simulink model "Kettle_System2_1"  (R2017b)
settings: Solver=VariableStepAuto  StartTime=0.0  StopTime=1000  FixedStep=1  MaxStep=1  RelTol=1e-3
libraries: simulink_extras x1
settings Model: DataTypeOverride=Double  MinMaxOverflowLogging=ForceOff  Creator=georgimarkov & jonhall  LastModifiedBy=georgimarkov

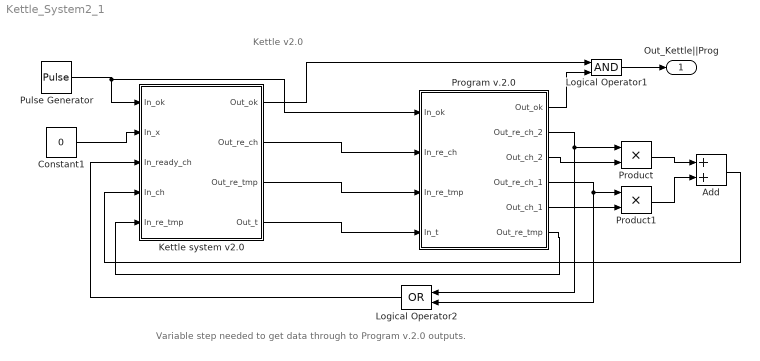
== system Kettle_System2_1 ==
  note: Variable step needed to get data through to Program v.2.0 outputs.
  note: Kettle v2.0
  Add : Sum
  Constant1 : Constant  Value=0
  Kettle system v2.0 : Subsystem
  Logical Operator1 : Logic  AllPortsSameDT=off  OutDataTypeStr=boolean
  Logical Operator2 : Logic  Operator=OR  AllPortsSameDT=off  OutDataTypeStr=boolean
  Product : Product
  Product1 : Product
  Program v.2.0 : Subsystem
  Pulse Generator : DiscretePulseGenerator  Period=200  PhaseDelay=10
  Out_Kettle||Prog : Outport
  wires:
  Program v.2.0/1(Out_ok) -> Logical Operator1/2
  Kettle system v2.0/1(Out_ok) -> Logical Operator1/1
  Logical Operator1/1 -> Out_Kettle||Prog/1
  Constant1/1 -> Kettle system v2.0/2(In_x)
  Kettle system v2.0/2(Out_re_ch) -> Program v.2.0/2(In_re_ch)
  Kettle system v2.0/3(Out_re_tmp) -> Program v.2.0/3(In_re_tmp)
  Program v.2.0/2(Out_re_ch_2) -> Logical Operator2/1, Product/1
  Program v.2.0/3(Out_ch_2) -> Product/2
  Program v.2.0/4(Out_re_ch_1) -> Logical Operator2/2, Product1/1
  Program v.2.0/5(Out_ch_1) -> Product1/2
  Product/1 -> Add/1
  Product1/1 -> Add/2
  Add/1 -> Kettle system v2.0/4(In_ch)
  Program v.2.0/6(Out_re_tmp) -> Kettle system v2.0/5(In_re_tmp)
  Logical Operator2/1 -> Kettle system v2.0/3(In_ready_ch)
  Kettle system v2.0/4(Out_t) -> Program v.2.0/4(In_t)
  Pulse Generator/1 -> Program v.2.0/1(In_ok), Kettle system v2.0/1(In_ok)

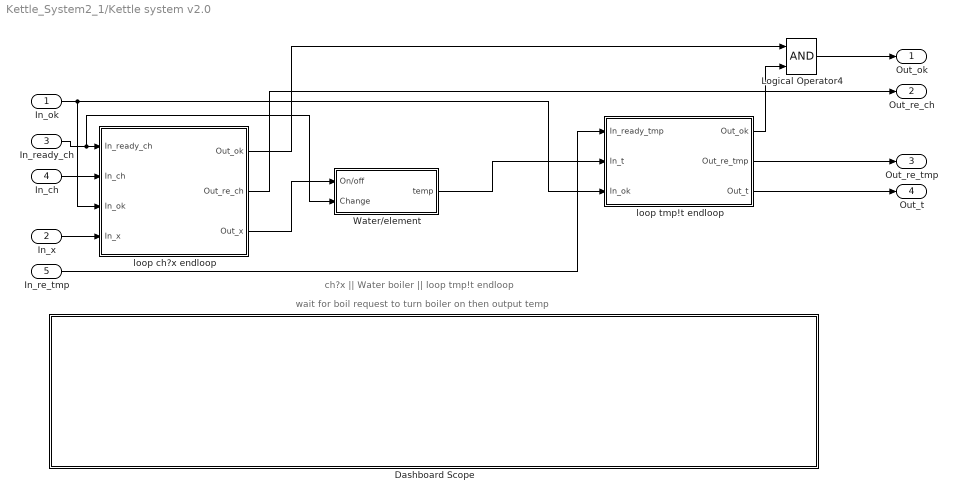
== system Kettle_System2_1/Kettle system v2.0 ==
  note: ch?x || Water boiler || loop tmp!t endloop
  note: wait for boil request to turn boiler on then output temp
  In_ok : Inport
  In_x : Inport  Port=2
  In_ready_ch : Inport  Port=3
  In_ch : Inport  Port=4
  In_re_tmp : Inport  Port=5
  Dashboard Scope : Subsystem  DialogController=hmiCreateDDGDialog  IsWebBlock=on  mask(MWDashboardBlock){webBlockId=0c6ab515-e131-4fbc-9890-d7af2ac4fa79, webBlockType=sdiscope, ShowInitialText=on, HMISrcModelName=Kettle_System2_1}
      mask prompts: webBlockId "WebBlock Id"; webBlockType "WebBlock Type"; HMISrcModelName "Source Model"
      mask help: SimulinkHMI:dialogs:HMIScopeDialogDesc
      mask Help: helpview([docroot '/mapfiles/simulink.map'], 'hmi_scope')
      mask Display:
      | if strcmp(get_param(bdroot(gcb),'BlockDiagramType'), 'library')
      |     image([(matlabroot) '/toolbox/simulink/hmi/icons/DashboardScope.png']);
      | end
  Logical Operator4 : Logic  AllPortsSameDT=off  OutDataTypeStr=fixdt(1,16)
  Water/element : Subsystem  TreatAsAtomicUnit=on  SystemSampleTime=0
  loop ch?x endloop : Subsystem
  loop tmp!t endloop : Subsystem
  Out_ok : Outport
  Out_re_ch : Outport  Port=2
  Out_re_tmp : Outport  Port=3
  Out_t : Outport  Port=4
  wires:
  Water/element/1(temp) -> loop tmp!t endloop/2(In_t)
  In_ok/1 -> loop tmp!t endloop/3(In_ok), loop ch?x endloop/3(In_ok)
  In_x/1 -> loop ch?x endloop/4(In_x)
  In_ready_ch/1 -> Water/element/2(Change), loop ch?x endloop/1(In_ready_ch)
  In_ch/1 -> loop ch?x endloop/2(In_ch)
  loop tmp!t endloop/1(Out_ok) -> Logical Operator4/2
  Logical Operator4/1 -> Out_ok/1
  In_re_tmp/1 -> loop tmp!t endloop/1(In_ready_tmp)
  loop tmp!t endloop/2(Out_re_tmp) -> Out_re_tmp/1
  loop tmp!t endloop/3(Out_t) -> Out_t/1
  loop ch?x endloop/1(Out_ok) -> Logical Operator4/1
  loop ch?x endloop/2(Out_re_ch) -> Out_re_ch/1
  loop ch?x endloop/3(Out_x) -> Water/element/1(On/off)

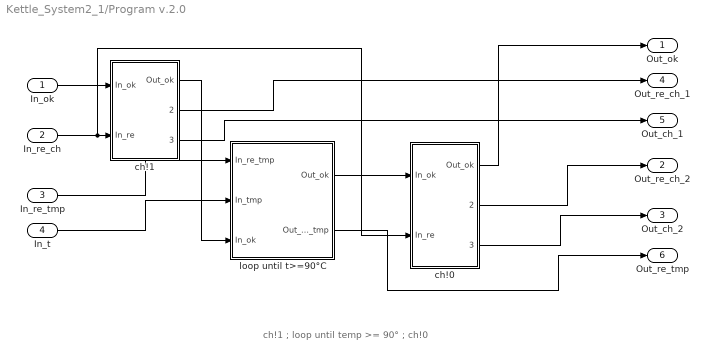
== system Kettle_System2_1/Program v.2.0 ==
  note: ch!1 ; loop until temp >= 90° ; ch!0
  In_ok : Inport
  In_re_ch : Inport  Port=2
  In_re_tmp : Inport  Port=3
  In_t : Inport  Port=4
  ch!0 : Subsystem
  "ch!1 " : Subsystem
  loop until t>=90°C : Subsystem
  Out_ok : Outport
  Out_re_ch_2 : Outport  Port=2
  Out_ch_2 : Outport  Port=3
  Out_re_ch_1 : Outport  Port=4
  Out_ch_1 : Outport  Port=5
  Out_re_tmp : Outport  Port=6
  wires:
  ch!0/2(Out_re_ch_2) -> Out_re_ch_2/1
  loop until t>=90°C/1(Out_ok) -> ch!0/1(In_ok)
  "ch!1 "/2(Out_re_ch_1) -> Out_re_ch_1/1
  "ch!1 "/1(Out_ok) -> loop until t>=90°C/3(In_ok)
  ch!0/1(Out_ok) -> Out_ok/1
  In_ok/1 -> "ch!1 "/1(In_ok)
  In_re_ch/1 -> ch!0/2(In_re), "ch!1 "/2(In_re)
  In_re_tmp/1 -> loop until t>=90°C/1(In_re_tmp)
  ch!0/3(Out_ch_2) -> Out_ch_2/1
  "ch!1 "/3("Out_ch_1 ") -> Out_ch_1/1
  loop until t>=90°C/2(Out_re_tmp) -> Out_re_tmp/1
  In_t/1 -> loop until t>=90°C/2(In_tmp)

== system Kettle_System2_1/Kettle system v2.0/Dashboard Scope ==

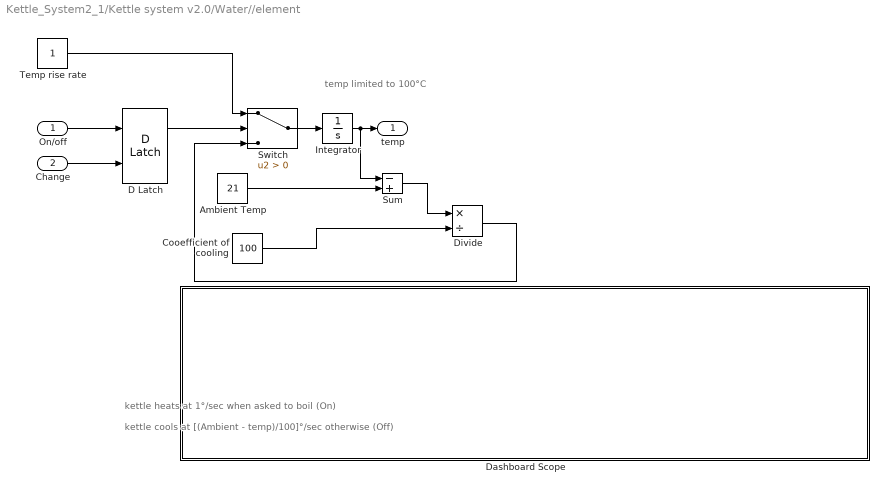
== system Kettle_System2_1/Kettle system v2.0/Water//element ==
  note: temp limited to 100°C
  note: kettle heats at 1°/sec when asked to boil (On)
  note: kettle cools at [(Ambient - temp)/100]°/sec otherwise (Off)
  On/off : Inport
  Change : Inport  Port=2
  "Ambient Temp " : Constant  Value=21
  Cooefficient of cooling : Constant  Value=100
  D Latch : simulink_extras/Flip Flops/D Latch
      settings: SourceProductName=Simulink  SourceProductBaseCode=SL
  Dashboard Scope : Subsystem  DialogController=hmiCreateDDGDialog  IsWebBlock=on  mask(MWDashboardBlock){webBlockId=a0783e22-3817-44e7-9254-d29470bf7746, webBlockType=sdiscope, ShowInitialText=on, HMISrcModelName=Kettle_System2_1}
      mask prompts: webBlockId "WebBlock Id"; webBlockType "WebBlock Type"; HMISrcModelName "Source Model"
      mask help: SimulinkHMI:dialogs:HMIScopeDialogDesc
      mask Help: helpview([docroot '/mapfiles/simulink.map'], 'hmi_scope')
      mask Display:
      | if strcmp(get_param(bdroot(gcb),'BlockDiagramType'), 'library')
      |     image([(matlabroot) '/toolbox/simulink/hmi/icons/DashboardScope.png']);
      | end
  Divide : Product  Inputs=*/
  Integrator : Integrator  InitialCondition=21  LimitOutput=on  UpperSaturationLimit=100  LowerSaturationLimit=-273.15
  Sum : Sum  Inputs=-+
  Switch : Switch  Criteria=u2 > Threshold
  Temp rise rate : Constant
  temp : Outport
  wires:
  Switch/1 -> Integrator/1
  Temp rise rate/1 -> Switch/1
  Divide/1 -> Switch/3
  D Latch/1 -> Switch/2
  Change/1 -> D Latch/2
  On/off/1 -> D Latch/1
  Integrator/1 -> Sum/1, temp/1
  Sum/1 -> Divide/1
  "Ambient Temp "/1 -> Sum/2
  Cooefficient of cooling/1 -> Divide/2

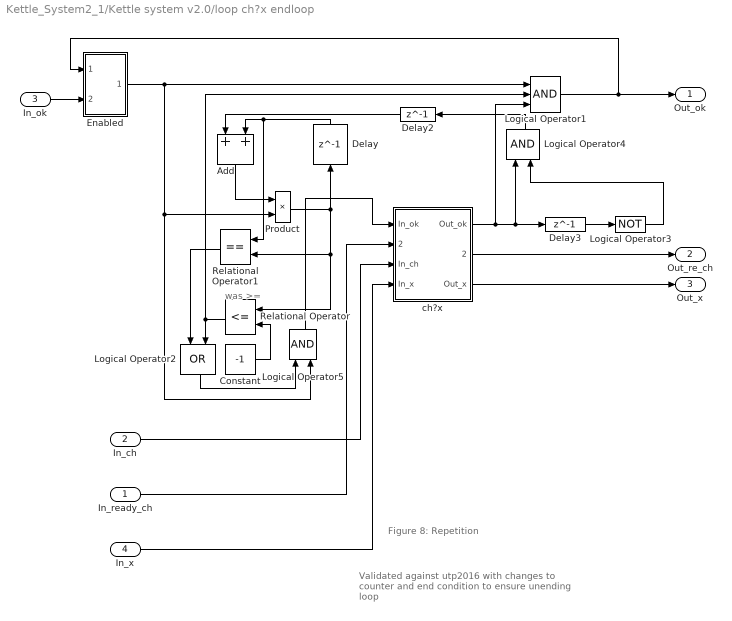
== system Kettle_System2_1/Kettle system v2.0/loop ch?x endloop ==
  note: was >=
  note: Figure 8: Repetition
  note: Validated against utp2016
      | with changes to counter and end condition to
      | ensure unending loop
  In_ready_ch : Inport
  In_ch : Inport  Port=2
  In_ok : Inport  Port=3
  In_x : Inport  Port=4
  Add : Sum
  Constant : Constant  Value=-1
  Delay : Delay  DelayLength=1  InitialCondition=0
  Delay2 : Delay  DelayLength=1  InitialCondition=0
  Delay3 : Delay  DelayLength=1  InitialCondition=0
  Enabled : Subsystem
  Logical Operator1 : Logic  Inputs=3  AllPortsSameDT=off  OutDataTypeStr=fixdt(1,16)
  Logical Operator2 : Logic  Operator=OR  AllPortsSameDT=off  OutDataTypeStr=fixdt(1,16)
  Logical Operator3 : Logic  Operator=NOT  AllPortsSameDT=off  OutDataTypeStr=fixdt(1,16)
  Logical Operator4 : Logic  AllPortsSameDT=off  OutDataTypeStr=fixdt(1,16)
  Logical Operator5 : Logic  AllPortsSameDT=off  OutDataTypeStr=fixdt(1,16)
  Product : Product
  Relational Operator : RelationalOperator  Operator=<=  OutDataTypeStr=boolean  RndMeth=Simplest
  Relational Operator1 : RelationalOperator  Operator===  OutDataTypeStr=boolean  RndMeth=Simplest
  ch?x : Subsystem
  Out_ok : Outport
  Out_re_ch : Outport  Port=2
  Out_x : Outport  Port=3
  wires:
  Enabled/1(Enabled) -> Logical Operator1/1, Product/2, Logical Operator5/2
  Logical Operator1/1 -> Enabled/1(Out_ok), Out_ok/1
  In_ch/1 -> ch?x/3(In_ch)
  Logical Operator4/1 -> Delay2/1
  Logical Operator2/1 -> Logical Operator5/1
  Delay3/1 -> Logical Operator3/1
  Constant/1 -> Relational Operator/2
  Delay2/1 -> Add/1
  Logical Operator3/1 -> Logical Operator4/2
  Delay/1 -> Add/2, Relational Operator1/1
  In_ready_ch/1 -> ch?x/2(In_re_ch)
  Add/1 -> Product/1
  Product/1 -> Relational Operator/1, Relational Operator1/2, Delay/1
  Logical Operator5/1 -> ch?x/1(In_ok)
  Relational Operator1/1 -> Logical Operator2/1
  Relational Operator/1 -> Logical Operator1/2, Logical Operator2/2
  In_ok/1 -> Enabled/2(In_ok)
  ch?x/1(Out_ok) -> Logical Operator4/1, Delay3/1, Logical Operator1/3
  ch?x/2(Out_re_ch) -> Out_re_ch/1
  ch?x/3("Out_x ") -> Out_x/1
  In_x/1 -> ch?x/4(In_x)

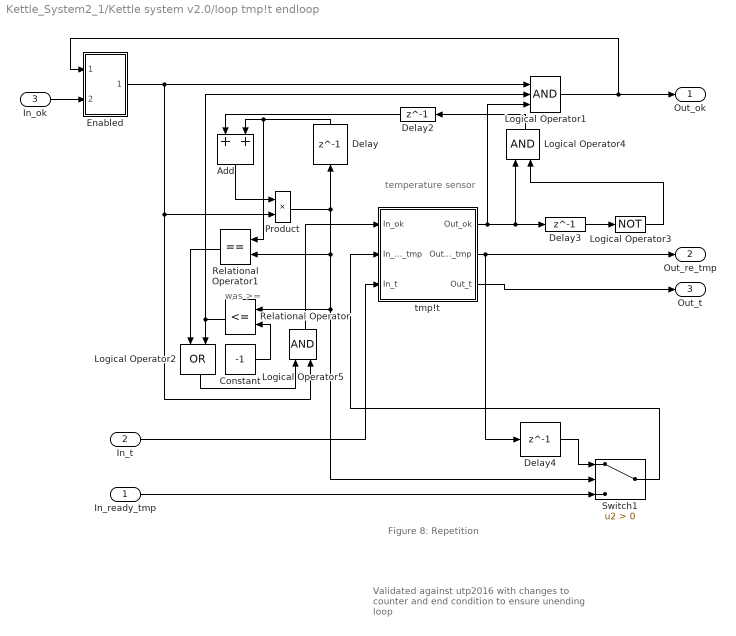
== system Kettle_System2_1/Kettle system v2.0/loop tmp!t endloop ==
  note: was >=
  note: Figure 8: Repetition
  note: temperature sensor
  note: Validated against utp2016
      | with changes to counter and end condition to
      | ensure unending loop
  In_ready_tmp : Inport
  In_t : Inport  Port=2
  In_ok : Inport  Port=3
  Add : Sum
  Constant : Constant  Value=-1
  Delay{,2..4} (4 alike) : Delay  DelayLength=1  InitialCondition=0
  Enabled : Subsystem
  Logical Operator1 : Logic  Inputs=3  AllPortsSameDT=off  OutDataTypeStr=fixdt(1,16)
  Logical Operator2 : Logic  Operator=OR  AllPortsSameDT=off  OutDataTypeStr=fixdt(1,16)
  Logical Operator3 : Logic  Operator=NOT  AllPortsSameDT=off  OutDataTypeStr=fixdt(1,16)
  Logical Operator4 : Logic  AllPortsSameDT=off  OutDataTypeStr=fixdt(1,16)
  Logical Operator5 : Logic  AllPortsSameDT=off  OutDataTypeStr=fixdt(1,16)
  Product : Product
  Relational Operator : RelationalOperator  Operator=<=  OutDataTypeStr=boolean  RndMeth=Simplest
  Relational Operator1 : RelationalOperator  Operator===  OutDataTypeStr=boolean  RndMeth=Simplest
  Switch1 : Switch  Criteria=u2 > Threshold  OutDataTypeStr=double
  tmp!t : Subsystem
  Out_ok : Outport
  Out_re_tmp : Outport  Port=2
  Out_t : Outport  Port=3
  wires:
  Enabled/1(Enabled) -> Logical Operator1/1, Product/2, Logical Operator5/2
  Logical Operator1/1 -> Enabled/1(Out_ok), Out_ok/1
  In_t/1 -> tmp!t/3(In_t)
  Logical Operator4/1 -> Delay2/1
  tmp!t/1(Out_ok) -> Delay3/1, Logical Operator4/1, Logical Operator1/3
  Logical Operator2/1 -> Logical Operator5/1
  Delay3/1 -> Logical Operator3/1
  Constant/1 -> Relational Operator/2
  tmp!t/2(Out_re_tmp) -> Out_re_tmp/1, Delay4/1
  Delay2/1 -> Add/1
  Logical Operator3/1 -> Logical Operator4/2
  Delay/1 -> Add/2, Relational Operator1/1
  In_ready_tmp/1 -> Switch1/3
  Delay4/1 -> Switch1/1
  Switch1/1 -> tmp!t/2(In_re_tmp)
  tmp!t/3("Out_t ") -> Out_t/1
  Add/1 -> Product/1
  Product/1 -> Relational Operator/1, Switch1/2, Relational Operator1/2, Delay/1
  Logical Operator5/1 -> tmp!t/1(In_ok)
  Relational Operator1/1 -> Logical Operator2/1
  Relational Operator/1 -> Logical Operator1/2, Logical Operator2/2
  In_ok/1 -> Enabled/2(In_ok)

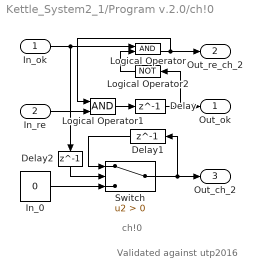
== system Kettle_System2_1/Program v.2.0/ch!0 ==
  note: Validated against utp2016
  note: ch!0
  In_ok : Inport
  In_re : Inport  Port=2
  Delay : Delay  DelayLength=1  InitialCondition=0
  Delay1 : Delay  DelayLength=1  InitialCondition=0
  Delay2 : Delay  DelayLength=1  InitialCondition=0
  "In_0 " : Constant  Value=0
  Logical Operator : Logic  AllPortsSameDT=off  OutDataTypeStr=fixdt(1,16)
  Logical Operator1 : Logic  AllPortsSameDT=off  OutDataTypeStr=fixdt(1,16)
  Logical Operator2 : Logic  Operator=NOT  AllPortsSameDT=off  OutDataTypeStr=fixdt(1,16)
  Switch : Switch  Criteria=u2 > Threshold
  Out_ok : Outport
  Out_re_ch_2 : Outport  Port=2
  Out_ch_2 : Outport  Port=3
  wires:
  In_re/1 -> Logical Operator1/2
  Logical Operator2/1 -> Logical Operator/2
  Logical Operator1/1 -> Delay/1
  In_ok/1 -> Logical Operator/1, Delay2/1
  Delay2/1 -> Switch/2
  Logical Operator/1 -> Out_re_ch_2/1, Logical Operator1/1
  Switch/1 -> Delay1/1, Out_ch_2/1
  Delay1/1 -> Switch/1
  "In_0 "/1 -> Switch/3
  Delay/1 -> Out_ok/1, Logical Operator2/1

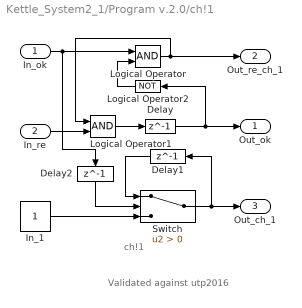
== system Kettle_System2_1/Program v.2.0/ch!1  ==
  note: Validated against utp2016
  note: ch!1
  In_ok : Inport
  In_re : Inport  Port=2
  Delay : Delay  DelayLength=1  InitialCondition=0
  Delay1 : Delay  DelayLength=1  InitialCondition=0
  Delay2 : Delay  DelayLength=1  InitialCondition=0
  In_1 : Constant
  Logical Operator : Logic  AllPortsSameDT=off  OutDataTypeStr=fixdt(1,16)
  Logical Operator1 : Logic  AllPortsSameDT=off  OutDataTypeStr=fixdt(1,16)
  Logical Operator2 : Logic  Operator=NOT  AllPortsSameDT=off  OutDataTypeStr=boolean
  Switch : Switch  Criteria=u2 > Threshold
  Out_ok : Outport
  Out_re_ch_1 : Outport  Port=2
  "Out_ch_1 " : Outport  Port=3
  wires:
  In_re/1 -> Logical Operator1/2
  Logical Operator2/1 -> Logical Operator/2
  In_ok/1 -> Delay2/1, Logical Operator/1
  Delay2/1 -> Switch/2
  Switch/1 -> Delay1/1, "Out_ch_1 "/1
  Delay1/1 -> Switch/1
  In_1/1 -> Switch/3
  Logical Operator/1 -> Out_re_ch_1/1, Logical Operator1/1
  Logical Operator1/1 -> Delay/1
  Delay/1 -> Logical Operator2/1, Out_ok/1

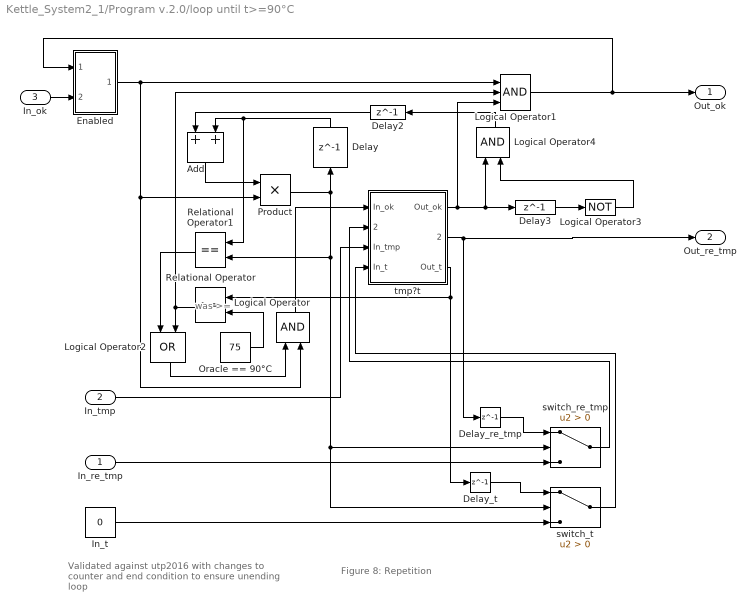
== system Kettle_System2_1/Program v.2.0/loop until t>=90°C ==
  note: Figure 8: Repetition
  note: was >=
  note: Validated against utp2016
      | with changes to counter and end condition to
      | ensure unending loop
  In_re_tmp : Inport
  In_tmp : Inport  Port=2
  In_ok : Inport  Port=3
  Add : Sum
  Delay : Delay  DelayLength=1  InitialCondition=0
  Delay2 : Delay  DelayLength=1  InitialCondition=0
  Delay3 : Delay  DelayLength=1  InitialCondition=0
  Delay_re_tmp : Delay  DelayLength=1  InitialCondition=0
  Delay_t : Delay  DelayLength=1  InitialCondition=0
  Enabled : Subsystem
  In_t : Constant  Value=0
  Logical Operator : Logic  AllPortsSameDT=off  OutDataTypeStr=boolean
  Logical Operator1 : Logic  Inputs=3  AllPortsSameDT=off  OutDataTypeStr=fixdt(1,16)
  Logical Operator2 : Logic  Operator=OR  AllPortsSameDT=off  OutDataTypeStr=fixdt(1,16)
  Logical Operator3 : Logic  Operator=NOT  AllPortsSameDT=off  OutDataTypeStr=fixdt(1,16)
  Logical Operator4 : Logic  AllPortsSameDT=off  OutDataTypeStr=fixdt(1,16)
  Oracle == 90°C : Constant  Value=75
  Product : Product
  Relational Operator : RelationalOperator  OutDataTypeStr=boolean  RndMeth=Simplest
  Relational Operator1 : RelationalOperator  Operator===  OutDataTypeStr=boolean  RndMeth=Simplest
  switch_re_tmp : Switch  Criteria=u2 > Threshold  OutDataTypeStr=double
  switch_t : Switch  Criteria=u2 > Threshold  OutDataTypeStr=double
  tmp?t : Subsystem
  Out_ok : Outport
  Out_re_tmp : Outport  Port=2
  wires:
  Enabled/1(Enabled) -> Logical Operator/2, Product/2, Logical Operator1/1
  In_tmp/1 -> tmp?t/3(In_tmp)
  Oracle == 90°C/1 -> Relational Operator/2
  Delay_t/1 -> switch_t/1
  Logical Operator3/1 -> Logical Operator4/2
  Logical Operator1/1 -> Enabled/1(Out_ok), Out_ok/1
  Relational Operator/1 -> Logical Operator2/2, Logical Operator1/2
  Delay/1 -> Add/2, Relational Operator1/1
  In_re_tmp/1 -> switch_re_tmp/3
  Logical Operator4/1 -> Delay2/1
  Delay2/1 -> Add/1
  tmp?t/3("Out_t ") -> Delay_t/1, Relational Operator/1
  tmp?t/1(Out_ok) -> Delay3/1, Logical Operator4/1, Logical Operator1/3
  Delay3/1 -> Logical Operator3/1
  tmp?t/2(Out_re_tmp) -> Out_re_tmp/1, Delay_re_tmp/1
  In_t/1 -> switch_t/3
  switch_re_tmp/1 -> tmp?t/2(In_re_tmp)
  switch_t/1 -> tmp?t/4(In_t)
  Delay_re_tmp/1 -> switch_re_tmp/1
  Relational Operator1/1 -> Logical Operator2/1
  Logical Operator2/1 -> Logical Operator/1
  Logical Operator/1 -> tmp?t/1(In_ok)
  Add/1 -> Product/1
  Product/1 -> switch_t/2, switch_re_tmp/2, Relational Operator1/2, Delay/1
  In_ok/1 -> Enabled/2(In_ok)

== system Kettle_System2_1/Kettle system v2.0/Water//element/Dashboard Scope ==

== system Kettle_System2_1/Kettle system v2.0/loop ch?x endloop/Enabled ==
  Out_ok : Inport
  In_ok : Inport  Port=2
  Delay : Delay  DelayLength=1  InitialCondition=0
  Delay1 : Delay  DelayLength=1  InitialCondition=0
  Logical Operator : Logic  Operator=OR  AllPortsSameDT=off  OutDataTypeStr=boolean
  Logical Operator1 : Logic  Operator=NOT  AllPortsSameDT=off  OutDataTypeStr=boolean
  Logical Operator2 : Logic  AllPortsSameDT=off  OutDataTypeStr=boolean
  Logical Operator3 : Logic  AllPortsSameDT=off  OutDataTypeStr=boolean
  Logical Operator4 : Logic  Operator=NOT  AllPortsSameDT=off  OutDataTypeStr=boolean
  Enabled : Outport
  wires:
  Logical Operator/1 -> Delay/1, Enabled/1
  Delay/1 -> Logical Operator3/2, Logical Operator1/1
  In_ok/1 -> Logical Operator2/1
  Logical Operator1/1 -> Logical Operator2/2
  Logical Operator2/1 -> Logical Operator/2
  Out_ok/1 -> Delay1/1
  Logical Operator3/1 -> Logical Operator/1
  Delay1/1 -> Logical Operator4/1
  Logical Operator4/1 -> Logical Operator3/1

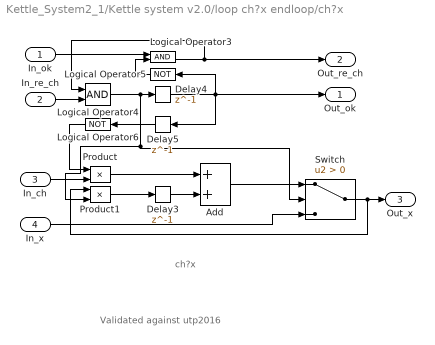
== system Kettle_System2_1/Kettle system v2.0/loop ch?x endloop/ch?x ==
  note: Validated against utp2016
  note: ch?x
  In_ok : Inport
  In_re_ch : Inport  Port=2
  In_ch : Inport  Port=3
  In_x : Inport  Port=4
  Add : Sum
  Delay3 : Delay  DelayLength=1  InitialCondition=0
  Delay4 : Delay  DelayLength=1  InitialCondition=0
  Delay5 : Delay  DelayLength=1  InitialCondition=0
  Logical Operator3 : Logic  AllPortsSameDT=off  OutDataTypeStr=fixdt(1,16)
  Logical Operator4 : Logic  AllPortsSameDT=off  OutDataTypeStr=fixdt(1,16)
  Logical Operator5 : Logic  Operator=NOT  AllPortsSameDT=off  OutDataTypeStr=fixdt(1,16)
  Logical Operator6 : Logic  Operator=NOT  AllPortsSameDT=off  OutDataTypeStr=fixdt(1,16)
  Product : Product
  Product1 : Product
  Switch : Switch  Criteria=u2 > Threshold
  Out_ok : Outport
  Out_re_ch : Outport  Port=2
  "Out_x " : Outport  Port=3
  wires:
  In_ch/1 -> Product/2
  In_ok/1 -> Logical Operator3/1
  Delay4/1 -> Out_ok/1, Delay5/1, Logical Operator5/1
  Product1/1 -> Delay3/1
  In_re_ch/1 -> Logical Operator4/2
  Logical Operator5/1 -> Logical Operator3/2
  Product/1 -> Add/1
  Delay3/1 -> Add/2
  Logical Operator6/1 -> Product/1
  Add/1 -> Switch/1
  Delay5/1 -> Logical Operator6/1
  Logical Operator3/1 -> Out_re_ch/1, Logical Operator4/1
  In_x/1 -> Switch/3
  Switch/1 -> "Out_x "/1, Product1/1
  Logical Operator4/1 -> Product1/2, Switch/2, Delay4/1

== system Kettle_System2_1/Kettle system v2.0/loop tmp!t endloop/Enabled ==
  Out_ok : Inport
  In_ok : Inport  Port=2
  Delay : Delay  DelayLength=1  InitialCondition=0
  Delay1 : Delay  DelayLength=1  InitialCondition=0
  Logical Operator : Logic  Operator=OR  AllPortsSameDT=off  OutDataTypeStr=boolean
  Logical Operator1 : Logic  Operator=NOT  AllPortsSameDT=off  OutDataTypeStr=boolean
  Logical Operator2 : Logic  AllPortsSameDT=off  OutDataTypeStr=boolean
  Logical Operator3 : Logic  AllPortsSameDT=off  OutDataTypeStr=boolean
  Logical Operator4 : Logic  Operator=NOT  AllPortsSameDT=off  OutDataTypeStr=boolean
  Enabled : Outport
  wires:
  Logical Operator/1 -> Delay/1, Enabled/1
  Delay/1 -> Logical Operator3/2, Logical Operator1/1
  In_ok/1 -> Logical Operator2/1
  Logical Operator1/1 -> Logical Operator2/2
  Logical Operator2/1 -> Logical Operator/2
  Out_ok/1 -> Delay1/1
  Logical Operator3/1 -> Logical Operator/1
  Delay1/1 -> Logical Operator4/1
  Logical Operator4/1 -> Logical Operator3/1

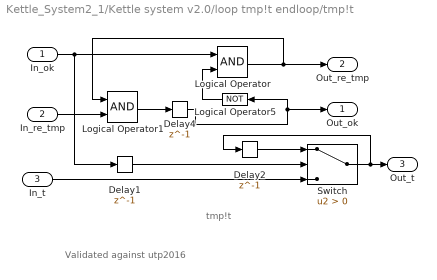
== system Kettle_System2_1/Kettle system v2.0/loop tmp!t endloop/tmp!t ==
  note: Validated against utp2016
  note: tmp!t
  In_ok : Inport
  In_re_tmp : Inport  Port=2
  In_t : Inport  Port=3
  Delay1 : Delay  DelayLength=1  InitialCondition=0
  Delay2 : Delay  DelayLength=1  InitialCondition=0
  Delay4 : Delay  DelayLength=1  InitialCondition=0
  Logical Operator : Logic  AllPortsSameDT=off  OutDataTypeStr=boolean
  Logical Operator1 : Logic  AllPortsSameDT=off  OutDataTypeStr=boolean
  Logical Operator5 : Logic  Operator=NOT  AllPortsSameDT=off  OutDataTypeStr=fixdt(1,16)
  Switch : Switch  Criteria=u2 > Threshold
  Out_ok : Outport
  Out_re_tmp : Outport  Port=2
  "Out_t " : Outport  Port=3
  wires:
  Switch/1 -> Delay2/1, "Out_t "/1
  In_t/1 -> Switch/3
  In_ok/1 -> Delay1/1, Logical Operator/1
  Logical Operator/1 -> Logical Operator1/1, Out_re_tmp/1
  Logical Operator5/1 -> Logical Operator/2
  In_re_tmp/1 -> Logical Operator1/2
  Logical Operator1/1 -> Delay4/1
  Delay4/1 -> Logical Operator5/1, Out_ok/1
  Delay1/1 -> Switch/2
  Delay2/1 -> Switch/1

== system Kettle_System2_1/Program v.2.0/loop until t>=90°C/Enabled ==
  Out_ok : Inport
  In_ok : Inport  Port=2
  Delay : Delay  DelayLength=1  InitialCondition=0
  Delay1 : Delay  DelayLength=1  InitialCondition=0
  Logical Operator : Logic  Operator=OR  AllPortsSameDT=off  OutDataTypeStr=boolean
  Logical Operator1 : Logic  Operator=NOT  AllPortsSameDT=off  OutDataTypeStr=boolean
  Logical Operator2 : Logic  AllPortsSameDT=off  OutDataTypeStr=boolean
  Logical Operator3 : Logic  AllPortsSameDT=off  OutDataTypeStr=boolean
  Logical Operator4 : Logic  Operator=NOT  AllPortsSameDT=off  OutDataTypeStr=boolean
  Enabled : Outport
  wires:
  Logical Operator/1 -> Delay/1, Enabled/1
  Delay/1 -> Logical Operator3/2, Logical Operator1/1
  In_ok/1 -> Logical Operator2/1
  Logical Operator1/1 -> Logical Operator2/2
  Logical Operator2/1 -> Logical Operator/2
  Out_ok/1 -> Delay1/1
  Logical Operator3/1 -> Logical Operator/1
  Delay1/1 -> Logical Operator4/1
  Logical Operator4/1 -> Logical Operator3/1

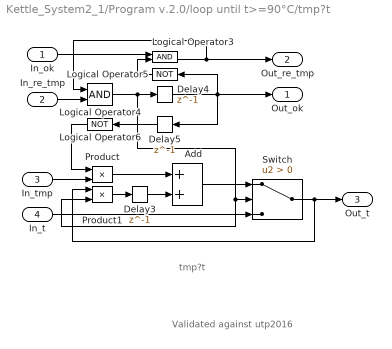
== system Kettle_System2_1/Program v.2.0/loop until t>=90°C/tmp?t ==
  note: Validated against utp2016
  note: tmp?t
  In_ok : Inport
  In_re_tmp : Inport  Port=2
  In_tmp : Inport  Port=3
  In_t : Inport  Port=4
  Add : Sum
  Delay3 : Delay  DelayLength=1  InitialCondition=0
  Delay4 : Delay  DelayLength=1  InitialCondition=0
  Delay5 : Delay  DelayLength=1  InitialCondition=0
  Logical Operator3 : Logic  AllPortsSameDT=off  OutDataTypeStr=fixdt(1,16)
  Logical Operator4 : Logic  AllPortsSameDT=off  OutDataTypeStr=fixdt(1,16)
  Logical Operator5 : Logic  Operator=NOT  AllPortsSameDT=off  OutDataTypeStr=fixdt(1,16)
  Logical Operator6 : Logic  Operator=NOT  AllPortsSameDT=off  OutDataTypeStr=fixdt(1,16)
  Product : Product
  Product1 : Product
  Switch : Switch  Criteria=u2 > Threshold
  Out_ok : Outport
  Out_re_tmp : Outport  Port=2
  "Out_t " : Outport  Port=3
  wires:
  In_tmp/1 -> Product/2
  In_ok/1 -> Logical Operator3/1
  Delay4/1 -> Out_ok/1, Delay5/1, Logical Operator5/1
  Product1/1 -> Delay3/1
  Logical Operator4/1 -> Product1/2, Switch/2, Delay4/1
  In_re_tmp/1 -> Logical Operator4/2
  Logical Operator5/1 -> Logical Operator3/2
  Product/1 -> Add/1
  Delay3/1 -> Add/2
  Logical Operator6/1 -> Product/1
  Add/1 -> Switch/1
  Delay5/1 -> Logical Operator6/1
  Logical Operator3/1 -> Out_re_tmp/1, Logical Operator4/1
  In_t/1 -> Switch/3
  Switch/1 -> "Out_t "/1, Product1/1
